simulink model "pid_controler"  (R2024b)
settings: Solver=VariableStepAuto  StartTime=0.0  StopTime=10.0  RelTol=1e-3
settings Model: Creator=user  LastModifiedBy=user

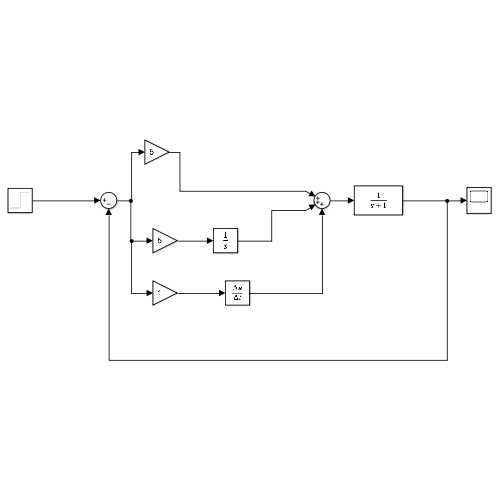
[thumbnail: Simulink's stored preview of the top-level diagram]
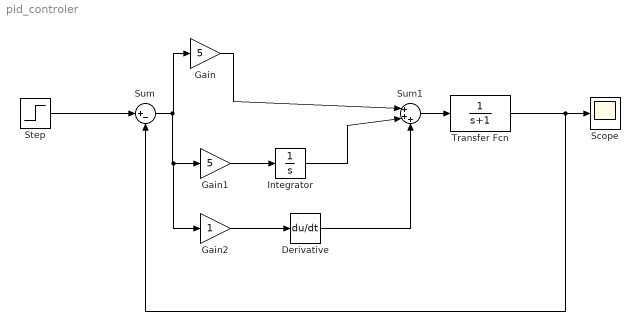
== system pid_controler ==
  Derivative : Derivative
  Gain : Gain  Gain=5
  Gain1 : Gain  Gain=5
  Gain2 : Gain
  Integrator : Integrator
  Scope : Scope
  Step : Step  SampleTime=0
  Sum : Sum  Inputs=|+-
  Sum1 : Sum  Inputs=|+++
  Transfer Fcn : TransferFcn  Denominator=[1 1]
  wires:
  Step/1 -> Sum/1
  Transfer Fcn/1 -> Sum/2, Scope/1
  Sum/1 -> Gain2/1, Gain1/1, Gain/1
  Gain/1 -> Sum1/1
  Gain1/1 -> Integrator/1
  Sum1/1 -> Transfer Fcn/1
  Integrator/1 -> Sum1/2
  Gain2/1 -> Derivative/1
  Derivative/1 -> Sum1/3
